simulink model "SynchronouslGenerater0"  (R2017b)
settings: Solver=ode3  StartTime=0.0  StopTime=7  MaxStep=1e-4  RelTol=1e-3  EnableMultiTasking=on
libraries: powerlib x27, powerlib_meascontrol x2
settings Model: Creator=1  LastModifiedBy=80573
settings DataIOCC: LimitDataPoints=on  SaveFormat=Array
settings OptimizationCC: LifeSpan=inf
settings DebuggingCC: SolverPrmCheckMsg=warning  SFUnexpectedBacktrackingDiag=warning  SFNoUnconditionalDefaultTransitionDiag=warning  SFExecutionAtInitializationDiag=none
settings HardwareCC: ProdBitPerPointer=32  ProdBitPerSizeT=32  ProdBitPerPtrDiffT=32  ProdLargestAtomicFloat=None  ProdIntDivRoundTo=Undefined  ProdEndianess=Unspecified  ProdWordSize=32  ProdHWDeviceType=32-bit Generic
settings ModelReferenceCC: PropagateSignalLabelsOutOfModel=off
settings CodeAppCC: StateflowObjectComments=on
settings GRTTargetCC: TargetLangStandard=C89/C90 (ANSI)  GeneratePreprocessorConditionals=Disable all
settings ConfigComp: CovMetricSettings=dw  CovHtmlReporting=on  CovSaveCumulativeToWorkspaceVar=on  CovSaveSingleToWorkspaceVar=on  CovExternalEMLEnable=off  CovSFcnEnable=off
settings SimscapeCC: SimscapeNormalizeSystem=off

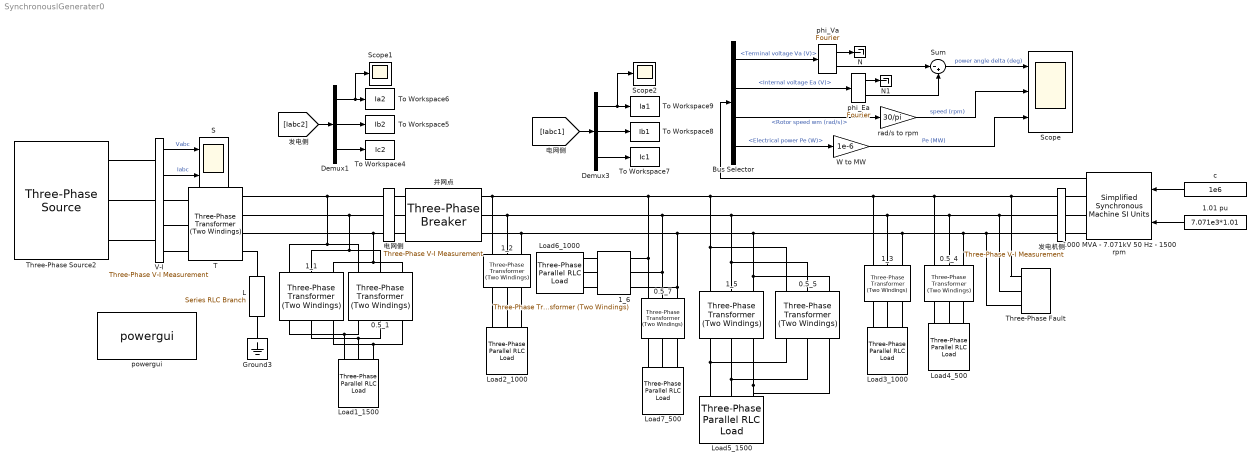
== system SynchronouslGenerater0 ==
  0.5_{1,4..5,7} (4 alike) : powerlib/Elements/Three-Phase Transformer (Two Windings)  Winding1Connection=Yg  Winding2Connection=Y  CoreType=Three single-phase transformers  SetSaturation=off  Hysteresis=off  DataFile='hysteresis'  SetInitialFlux=off  Measurements=None  UNITS=pu  NominalPower=[ 0.5e6 , 50 ]  Winding1=[7.071e3 0 0]  Winding2=[0.2828e3 10.2e-3 0.04]  Rm=744  Lm=333  L0=0.5  Saturation=[0 0;0.10998 5.4558;45.824 6.9106]  InitialFluxes=[3.6371 -3.6371 3.1824]  MoreParameters=off  BreakLoop=off  DataType=off  TransfoNumber=1
  1.01 pu : Constant  Value=7.071e3*1.01
  1000 MVA - 7.071kV 50 Hz - 1500 rpm : powerlib/Machines/Simplified Synchronous Machine SI Units  ConnectionType=3-wire Y  MechanicalLoad=Mechanical power Pm  MeasurementBus=off  NominalParameters=[ 1e6, 7.071e3, 50 ]  Mechanical="[1688,  200,  2]"  InternalRL=[ 49.999*0.02 ,49.999/(2*pi*50)*0.2 ]  InitialConditions=[0 6 0 0 0 0 -120 120]  Units=1  LoadFlowParameters=[1 500000000 0 0 0]  TsPowergui=0  TsBlock=-1  BusType=PV  Pref=0  Qref=0  Qmin=-inf  Qmax=+inf  PLF=0  QLF=0
      settings: AttributesFormatString=\n  SourceProductName=Simscape Power Systems  SourceProductBaseCode=PS
  1_{1..3,5..6} (5 alike) : powerlib/Elements/Three-Phase Transformer (Two Windings)  Winding1Connection=Yg  Winding2Connection=Y  CoreType=Three single-phase transformers  SetSaturation=off  Hysteresis=off  DataFile='hysteresis'  SetInitialFlux=off  Measurements=None  UNITS=pu  NominalPower=[ 1e6 , 50 ]  Winding1=[7.071e3 0 0]  Winding2=[0.2828e3 13.7e-3 55.3e-3]  Rm=6.9  Lm=58.4  L0=0.5  Saturation=[0 0;0.10998 5.4558;45.824 6.9106]  InitialFluxes=[3.6371 -3.6371 3.1824]  MoreParameters=off  BreakLoop=off  DataType=off  TransfoNumber=1
  Bus Selector : BusSelector  OutputSignals=Terminal voltage Va (V),Internal voltage Ea (V),Rotor speed wm (rad/s),Electrical power Pe (W)
  Demux1 : Demux  Outputs=3
  Demux3 : Demux  Outputs=3
  Ground3 : powerlib/Elements/Ground  LConnTagsString=a
  L : powerlib/Elements/Series RLC Branch  LConnTagsString=__new0  RConnTagsString=__new0  BranchType=L  Resistance=6  Inductance=0.283  SetiL0=off  InitialCurrent=0  Capacitance=1e-6  Setx0=off  InitialVoltage=0  Measurements=None
  Load1_1500 : powerlib/Elements/Three-Phase Parallel RLC Load  LConnTagsString=A|B|C  Configuration=Y (grounded)  NominalVoltage=282.8  Vabc=[1e3 1e3 1e3]  Vabcp=[1e3 1e3 1e3]  NominalFrequency=50  UnbalancedPower=off  ActivePower=240e3  InductivePower=180e3  CapacitivePower=0  Pabc=[10e3 9e3 11e3]  QLabc=[100 90 110]  QCabc=[100 90 110]  Pabcp=[10e3 9e3 11e3]  QLabcp=[100 90 110]  QCabcp=[100 90 110]  Measurements=None  LoadType=constant Z
  Load2_1000 : powerlib/Elements/Three-Phase Parallel RLC Load  LConnTagsString=A|B|C  Configuration=Y (grounded)  NominalVoltage=282.8  Vabc=[1e3 1e3 1e3]  Vabcp=[1e3 1e3 1e3]  NominalFrequency=50  UnbalancedPower=off  ActivePower=160e3  InductivePower=120e3  CapacitivePower=0  Pabc=[10e3 9e3 11e3]  QLabc=[100 90 110]  QCabc=[100 90 110]  Pabcp=[10e3 9e3 11e3]  QLabcp=[100 90 110]  QCabcp=[100 90 110]  Measurements=None  LoadType=constant Z
  Load3_1000 : powerlib/Elements/Three-Phase Parallel RLC Load  LConnTagsString=A|B|C  Configuration=Y (grounded)  NominalVoltage=282.8  Vabc=[1e3 1e3 1e3]  Vabcp=[1e3 1e3 1e3]  NominalFrequency=50  UnbalancedPower=off  ActivePower=160e3  InductivePower=120e3  CapacitivePower=0  Pabc=[10e3 9e3 11e3]  QLabc=[100 90 110]  QCabc=[100 90 110]  Pabcp=[10e3 9e3 11e3]  QLabcp=[100 90 110]  QCabcp=[100 90 110]  Measurements=None  LoadType=constant Z
  Load4_500 : powerlib/Elements/Three-Phase Parallel RLC Load  LConnTagsString=A|B|C  Configuration=Y (grounded)  NominalVoltage=282.8  Vabc=[1e3 1e3 1e3]  Vabcp=[1e3 1e3 1e3]  NominalFrequency=50  UnbalancedPower=off  ActivePower=80e3  InductivePower=60e3  CapacitivePower=0  Pabc=[10e3 9e3 11e3]  QLabc=[100 90 110]  QCabc=[100 90 110]  Pabcp=[10e3 9e3 11e3]  QLabcp=[100 90 110]  QCabcp=[100 90 110]  Measurements=None  LoadType=constant Z
  Load5_1500 : powerlib/Elements/Three-Phase Parallel RLC Load  LConnTagsString=A|B|C  Configuration=Y (grounded)  NominalVoltage=282.8  Vabc=[1e3 1e3 1e3]  Vabcp=[1e3 1e3 1e3]  NominalFrequency=50  UnbalancedPower=off  ActivePower=240e3  InductivePower=180e3  CapacitivePower=0  Pabc=[10e3 9e3 11e3]  QLabc=[100 90 110]  QCabc=[100 90 110]  Pabcp=[10e3 9e3 11e3]  QLabcp=[100 90 110]  QCabcp=[100 90 110]  Measurements=None  LoadType=constant Z
  Load6_1000 : powerlib/Elements/Three-Phase Parallel RLC Load  LConnTagsString=A|B|C  Configuration=Y (grounded)  NominalVoltage=282.8  Vabc=[1e3 1e3 1e3]  Vabcp=[1e3 1e3 1e3]  NominalFrequency=50  UnbalancedPower=off  ActivePower=160e3  InductivePower=120e3  CapacitivePower=0  Pabc=[10e3 9e3 11e3]  QLabc=[100 90 110]  QCabc=[100 90 110]  Pabcp=[10e3 9e3 11e3]  QLabcp=[100 90 110]  QCabcp=[100 90 110]  Measurements=None  LoadType=constant Z
  Load7_500 : powerlib/Elements/Three-Phase Parallel RLC Load  LConnTagsString=A|B|C  Configuration=Y (grounded)  NominalVoltage=282.8  Vabc=[1e3 1e3 1e3]  Vabcp=[1e3 1e3 1e3]  NominalFrequency=50  UnbalancedPower=off  ActivePower=80e3  InductivePower=60e3  CapacitivePower=0  Pabc=[10e3 9e3 11e3]  QLabc=[100 90 110]  QCabc=[100 90 110]  Pabcp=[10e3 9e3 11e3]  QLabcp=[100 90 110]  QCabcp=[100 90 110]  Measurements=None  LoadType=constant Z
  N : Terminator
  N1 : Terminator
  S : Scope  NumInputPorts=2
  Scope : Scope  NumInputPorts=3
  Scope1 : Scope
  Scope2 : Scope
  Sum : Sum  Inputs=|-+  SaturateOnIntegerOverflow=on  InputSameDT=on  OutDataTypeStr=Inherit: Same as first input
  T : powerlib/Elements/Three-Phase Transformer (Two Windings)  Winding1Connection=Yg  Winding2Connection=Yn  CoreType=Three single-phase transformers  SetSaturation=off  Hysteresis=off  DataFile='hysteresis'  SetInitialFlux=off  Measurements=None  UNITS=pu  NominalPower=[31.5e6 , 50 ]  Winding1=[77.782e3 0 0]  Winding2=[7.071e3 6e-3 104.8e-3]  Rm=22  Lm=148.4  L0=0.5  Saturation=[0 0;0.0034913 5.4558;1.4547 6.9106]  InitialFluxes=[3.6371 -3.6371 3.1824]  MoreParameters=off  BreakLoop=off  DataType=off  TransfoNumber=1
  Three-Phase Fault : powerlib/Elements/Three-Phase Fault  InitialStates=0  FaultA=on  FaultB=on  FaultC=on  GroundFault=on  SwitchTimes="[3  3+1/50]"  External=off  SwitchStatus=NaN  FaultResistance=0.001  GroundResistance=0.01  SnubberResistance=1e6  SnubberCapacitance=inf  Measurements=None
  Three-Phase Source2 : powerlib/Electrical Sources/Three-Phase Source  InternalConnection=Yg  VoltagePhases=off  Voltage=(77782)*1.00008  PhaseAngle=0.014178  Voltage_phases=[25e3 25e3 25e3]/sqrt(3)  PhaseAngles_phases=[0 -120 +120]  Frequency=50  NonIdealSource=on  SpecifyImpedance=off  Resistance=0.0929  Inductance=1.658e-3  ShortCircuitLevel=100e6  BaseVoltage=77.782e3  XRratio=7  BusType=swing  Pref=0  Qref=0  Prefabc=[10e3, 10e3, 10e3]  Qrefabc=[0, 0, 0]  Qmin=-inf  Qmax=inf
  To Workspace4 : ToWorkspace  VariableName=Ic2  SaveFormat=Timeseries  SampleTime=-1
  To Workspace5 : ToWorkspace  VariableName=Ib2  SaveFormat=Timeseries  SampleTime=-1
  To Workspace6 : ToWorkspace  VariableName=Ia2  SaveFormat=Timeseries  SampleTime=-1
  To Workspace7 : ToWorkspace  VariableName=Ic1  SaveFormat=Timeseries  SampleTime=-1
  To Workspace8 : ToWorkspace  VariableName=Ib1  SaveFormat=Timeseries  SampleTime=-1
  To Workspace9 : ToWorkspace  VariableName=Ia1  SaveFormat=Timeseries  SampleTime=-1
  V-I : powerlib/Measurements/Three-Phase V-I Measurement  VoltageMeasurement=phase-to-ground  SetLabelV=off  LabelV=Vabc  Vpu=off  VpuLL=off  CurrentMeasurement=yes  SetLabelI=off  LabelI=Iabc  Ipu=off  Pbase=100e6  Vbase=500e3  OutputType=Complex  PhasorSimulation=off  PSBequivalent=0
  W to MW : Gain  Gain=1e-6  SaturateOnIntegerOverflow=on  OutDataTypeStr=Inherit: Same as input  ParamDataTypeStr=Inherit: Same as input
  c : Constant  Value=1e6
  phi_Ea : powerlib_meascontrol/Measurements/Fourier  Freq=50  n=1  InInit=[0, 0]  Ts=0
      settings: SourceProductName=Simscape Power Systems
  phi_Va : powerlib_meascontrol/Measurements/Fourier  Freq=50  n=1  InInit=[0, 0]  Ts=0
      settings: SourceProductName=Simscape Power Systems
  powergui : powerlib/powergui  Priority=1  SimulationMode=Discrete  SampleTime=1e-4  frequency=60  Iterations=50  frequencyindice=50  Pbase=100e6  ErrMax=1e-4  UnitsV=kV  UnitsW=MW  buscounter=0  FunctionMessages=off  echomessages=off  EnableUseOfTLC=off  CurrentSourceSwitches=off  DisableSnubberDevices=off  DisableRonSwitches=off  DisableVfSwitches=off  DisplayEquations=off  SolverType=Tustin/Backward Euler (TBE)  Interpol=off  ExternalGateDelay=off  methode=off  Ts=100  x0status=blocks  SPID=on  SwTol=0  HookPort=off  RestoreLinks=warning  ResistiveCurrentMeasurement=off  Frange=[0:2:500]  Ylog=off  Xlog=on  ShowGrid=off  save=off  variable=ZData  structure=0  ZoomFFT=off  StartTime=0.0  cycles=1  DisplayStyle=1  fundamental=60  FreqAxis=off  MaxFrequency=1000  frequencyindicesteady=1  RmsSteady=1  display=off
  rad/s to rpm : Gain  Gain=30/pi  SaturateOnIntegerOverflow=on  OutDataTypeStr=Inherit: Same as input  ParamDataTypeStr=Inherit: Same as input
  发电机侧 : powerlib/Measurements/Three-Phase V-I Measurement  VoltageMeasurement=phase-to-ground  SetLabelV=on  LabelV=Vabc2  Vpu=off  VpuLL=off  CurrentMeasurement=yes  SetLabelI=on  LabelI=Iabc2  Ipu=off  Pbase=100e6  Vbase=500e3  OutputType=Complex  PhasorSimulation=off  PSBequivalent=0
  并网点 : powerlib/Elements/Three-Phase Breaker  InitialState=closed  SwitchA=on  SwitchB=on  SwitchC=on  SwitchTimes=[2 4]  External=off  BreakerResistance=0.01  SnubberResistance=1e6  SnubberCapacitance=1e-12  Measurements=None
  电网侧 : powerlib/Measurements/Three-Phase V-I Measurement  VoltageMeasurement=phase-to-ground  SetLabelV=on  LabelV=Vabc1  Vpu=off  VpuLL=off  CurrentMeasurement=yes  SetLabelI=on  LabelI=Iabc1  Ipu=off  Pbase=100e6  Vbase=500e3  OutputType=Complex  PhasorSimulation=off  PSBequivalent=0
  wires:
  Demux3/3 -> To Workspace7/1
  [Iabc1] -> Demux3/1
  Demux3/1 -> Scope2/1, To Workspace9/1
  Demux3/2 -> To Workspace8/1
  Sum/1 -> Scope/1  "power angle delta (deg)"
  Demux1/1 -> Scope1/1, To Workspace6/1
  phi_Va/1 -> N/1
  V-I/2 -> S/2  "Iabc"
  [Iabc2] -> Demux1/1
  Demux1/3 -> To Workspace4/1
  W to MW/1 -> Scope/3  "Pe (MW)"
  rad/s to rpm/1 -> Scope/2  "speed (rpm)"
  phi_Ea/1 -> N1/1
  phi_Va/2 -> Sum/1
  Bus Selector/3 -> rad/s to rpm/1  "<Rotor speed wm (rad/s)>"
  Bus Selector/4 -> W to MW/1  "<Electrical power Pe (W)>"
  Bus Selector/2 -> phi_Ea/1  "<Internal voltage Ea (V)>"
  Demux1/2 -> To Workspace5/1
  1000 MVA - 7.071kV 50 Hz - 1500 rpm/1 -> Bus Selector/1
  c/1 -> 1000 MVA - 7.071kV 50 Hz - 1500 rpm/1
  phi_Ea/2 -> Sum/2
  V-I/1 -> S/1  "Vabc"
  1.01 pu/1 -> 1000 MVA - 7.071kV 50 Hz - 1500 rpm/2
  Bus Selector/1 -> phi_Va/1  "<Terminal voltage Va (V)>"
  connections:
  0.5_4/LConn1 -- Three-Phase Fault/LConn1 -- 发电机侧/LConn1 -- 1_3/LConn1 -- 并网点/RConn1 -- 1_2/LConn1 -- 1_6/LConn1 -- 0.5_7/LConn1 -- 1_5/LConn1 -- 0.5_5/LConn1
  0.5_1/RConn2 -- 1_1/RConn2 -- Load1_1500/LConn2
  1_5/LConn3 -- 0.5_7/LConn3 -- 1_6/LConn3 -- 1_2/LConn3 -- 并网点/RConn3 -- 1_3/LConn3 -- Three-Phase Fault/LConn3 -- 发电机侧/LConn3 -- 0.5_4/LConn3 -- 0.5_5/LConn3
  电网侧/LConn2 -- T/RConn2 -- 0.5_1/LConn2 -- 1_1/LConn2
  0.5_4/LConn2 -- Three-Phase Fault/LConn2 -- 发电机侧/LConn2 -- 1_3/LConn2 -- 0.5_5/LConn2 -- 1_5/LConn2 -- 1_6/LConn2 -- 0.5_7/LConn2 -- 1_2/LConn2 -- 并网点/RConn2
  T/RConn3 -- 1_1/LConn3 -- 0.5_1/LConn3 -- 电网侧/LConn3
  0.5_5/RConn2 -- 1_5/RConn2 -- Load5_1500/LConn2
  T/RConn1 -- 电网侧/LConn1 -- 0.5_1/LConn1 -- 1_1/LConn1
  0.5_1/RConn1 -- 1_1/RConn1 -- Load1_1500/LConn1
  0.5_1/RConn3 -- 1_1/RConn3 -- Load1_1500/LConn3
  0.5_5/RConn1 -- 1_5/RConn1 -- Load5_1500/LConn1
  0.5_5/RConn3 -- 1_5/RConn3 -- Load5_1500/LConn3
  V-I/RConn1 -- T/LConn1
  Load7_500/LConn2 -- 0.5_7/RConn2
  Ground3/LConn1 -- L/LConn1
  Three-Phase Source2/RConn1 -- V-I/LConn1
  电网侧/RConn2 -- 并网点/LConn2
  Load3_1000/LConn2 -- 1_3/RConn2
  Three-Phase Source2/RConn2 -- V-I/LConn2
  V-I/RConn3 -- T/LConn3
  Three-Phase Source2/RConn3 -- V-I/LConn3
  发电机侧/RConn3 -- 1000 MVA - 7.071kV 50 Hz - 1500 rpm/RConn3
  发电机侧/RConn1 -- 1000 MVA - 7.071kV 50 Hz - 1500 rpm/RConn1
  1_2/RConn1 -- Load2_1000/LConn1
  发电机侧/RConn2 -- 1000 MVA - 7.071kV 50 Hz - 1500 rpm/RConn2
  Load2_1000/LConn2 -- 1_2/RConn2
  电网侧/RConn1 -- 并网点/LConn1
  1_2/RConn3 -- Load2_1000/LConn3
  Load4_500/LConn2 -- 0.5_4/RConn2
  1_6/RConn1 -- Load6_1000/LConn1
  1_3/RConn3 -- Load3_1000/LConn3
  1_3/RConn1 -- Load3_1000/LConn1
  Load6_1000/LConn2 -- 1_6/RConn2
  V-I/RConn2 -- T/LConn2
  电网侧/RConn3 -- 并网点/LConn3
  0.5_7/RConn3 -- Load7_500/LConn3
  L/RConn1 -- T/RConn4
  1_6/RConn3 -- Load6_1000/LConn3
  0.5_7/RConn1 -- Load7_500/LConn1
  0.5_4/RConn3 -- Load4_500/LConn3
  0.5_4/RConn1 -- Load4_500/LConn1
